simulink model "controllo_Completo_v14"  (R2025a)
settings: Solver=VariableStepAuto  StartTime=0.0  StopTime=Durata_Simulazione  MaxStep=Passo_integrazione_massimo  RelTol=1e-3
values from neighbouring files (symbols this model uses):
  C_bat_eq_rx = 1.0    (= 1)    [p_schema_completo_generale_v2.m]
  C_bat_eq_tx = 3.5    [p_schema_completo_generale_v2.m]
  C_bus_dc_dc = 1.5e-3    (= 0.0015)    [p_schema_completo_generale_v2.m]
  C_ris = 1/(w_dc_ac_nom^2*L_coil)    (= 6.49245057301e-08)    [p_schema_completo_generale_v2.m]
  dead_time_dc_dc = 0.3e-6    (= 3e-07)    [p_schema_completo_generale_v2.m]
  duty_A_0_tx = V_bat_0_tx/V_dc_0_tx    (= 0.472727272727)    [p_schema_completo_generale_v2.m]
  duty_B_0_tx = duty_A_0_tx    (= 0.472727272727)    [p_schema_completo_generale_v2.m]
  duty_leg_A_dc_dc_0_tx = V_bat_0_tx/V_dc_0_tx    (= 0.472727272727)    [p_schema_completo_generale_v2.m]
  duty_leg_B_dc_dc_0_tx = duty_leg_A_dc_dc_0_tx    (= 0.472727272727)    [p_schema_completo_generale_v2.m]
  Ibat_rif_max = 50    [p_schema_completo_generale_v2.m]
  Ibat_rif_min = -50    [p_schema_completo_generale_v2.m]
  Kp_P_tensione_batteria_rx = 1/modulo_catena_aperta_tensione_batteria_reg_P_rx    [p_schema_completo_generale_v2.m]
  Kp_P_tensione_batteria_tx = 1/modulo_catena_aperta_tensione_batteria_reg_P_tx    [p_schema_completo_generale_v2.m]
  L_coil = 54e-6    (= 5.4e-05)    [p_schema_completo_generale_v2.m]
  L_filtro_dc_dc = 65e-6    (= 6.5e-05)    [p_schema_completo_generale_v2.m]
  M_coil = k*sqrt(L_coil^2)    [p_schema_completo_generale_v2.m]
  Parametri_Controllori = [Parametri_Controllori     PI_corrente_trasm_tf_disc_den(2) PI_corrente_trasm_tf_disc_num(1) PI_corrente_trasm_tf_disc_num(2)]    [p_schema_completo_generale_v2.m]
  R_bat = 32e-3    (= 0.032)    [p_schema_completo_generale_v2.m]
  R_coil = w_dc_ac_nom*L_coil/Q_coil    (= 0.2883982056)    [p_schema_completo_generale_v2.m]
  R_coil_M = sqrt(w_dc_ac_nom^2)*M_coil/sqrt(Q_coil^2)    [p_schema_completo_generale_v2.m]
  R_Lfiltro_dc_dc = 6.5e-3    (= 0.0065)    [p_schema_completo_generale_v2.m]
  Req_Lfiltro_dc_dc = (R_Lfiltro_dc_dc+Rds_on_dc_dc)    (= 0.0075)    [p_schema_completo_generale_v2.m]
  Rshunt_coil = 1e5    (= 100000)    [p_schema_completo_generale_v2.m]
  Rshunt_Lfiltro = 1e6    (= 1000000)    [p_schema_completo_generale_v2.m]
  T_dc_ac = 1/freq_dc_ac    (= 1.17647058824e-05)    [p_schema_completo_generale_v2.m]
  T_dc_dc = 1/freq_dc_dc    (= 7.8431372549e-06)    [p_schema_completo_generale_v2.m]
  tau_filtro_anti_aliasing = R_filtro_anti_aliasing*C_filtro_anti_aliasing    (= 1.96e-06)    [p_schema_completo_generale_v2.m]
  tau_filtro_pb_coil = 1/(2*pi*f_filtro_pb_coil)    (= 3.18309886184e-05)    [p_schema_completo_generale_v2.m]
  tau_filtro_pb_corrente_bat = 1/(2*pi*f_filtro_pb_corrente_bat)    (= 2.49654812693e-05)    [p_schema_completo_generale_v2.m]
  Ts_BMS = 1e-3    (= 0.001)    [p_schema_completo_generale_v2.m]
  Ts_dc_ac = 4*T_dc_ac    (= 4.70588235294e-05)    [p_schema_completo_generale_v2.m]
  Ts_dc_dc = Ts_dc_ac    (= 4.70588235294e-05)    [p_schema_completo_generale_v2.m]
  Ts_trasmissione = 1e-3    (= 0.001)    [p_schema_completo_generale_v2.m]
  V_bat_0_rx = V_bat_nom    (= 96)    [p_schema_completo_generale_v2.m]
  V_bat_0_tx = V_bat_max-5    (= 104)    [p_schema_completo_generale_v2.m]
  V_bat_max = 109    [p_schema_completo_generale_v2.m]
  V_bat_max_alg = 218    [Controllo_tensione_bus_dc.m]    (also in Controllo_tensione_bus_dc_corrente_bobina.m; p_schema_completo_generale_v2.m)
  V_bat_min = 75    [p_schema_completo_generale_v2.m]
  V_bat_min_alg = 37.5    [Controllo_tensione_bus_dc.m]    (also in Controllo_tensione_bus_dc_corrente_bobina.m; p_schema_completo_generale_v2.m)
  V_dc_0_rx = 230    [p_schema_completo_generale_v2.m]
  V_dc_0_tx = 220    [p_schema_completo_generale_v2.m]
  Vbat_rif_max_tx = V_bat_max    (= 109)    [p_schema_completo_generale_v2.m]
  Vbat_rif_min_tx = V_bat_min    (= 75)    [p_schema_completo_generale_v2.m]
  Vdc_rif_max_tx = V_dc_nom+5    (= 255)    [p_schema_completo_generale_v2.m]
  Vdc_rif_min_tx = V_dc_nom-5    (= 245)    [p_schema_completo_generale_v2.m]
undefined symbols (not defined in the file or in its folder): Ceq_bat_tx, Cris_tx, Lfilt_dc_dc, Lfiltro_dc_dc_tx, R_bat_rx, R_bat_tx
libraries: simulink x44, spsSeriesRLCBranchLib x36, spsCurrentMeasurementLib x20, spsMosfetLib x16, spsVoltageMeasurementLib x12, simulink_extras x4, spsControlledCurrentSourceLib x4, spsControlledVoltageSourceLib x4, spsDCVoltageSourceLib x2, spsMutualInductanceLib x1, spsGroundLib x1, sps_lib x1
(part 1 of 7)
settings Model: Creator=bertman38930  LastModifiedBy=bertman38930
settings SolverCC: ZeroCrossAlgorithm=Adaptive
settings DebuggingCC: IgnoredZcDiagnostic=none

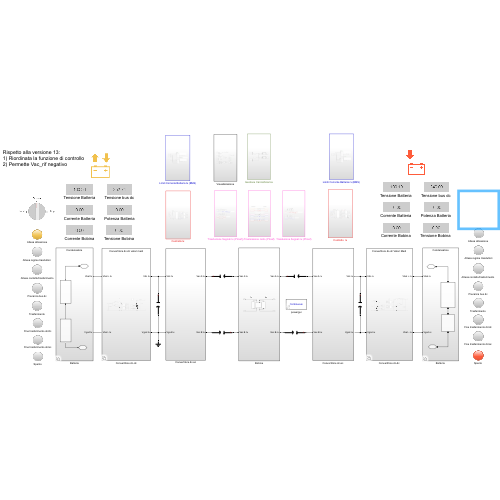
[thumbnail: Simulink's stored preview of the top-level diagram]
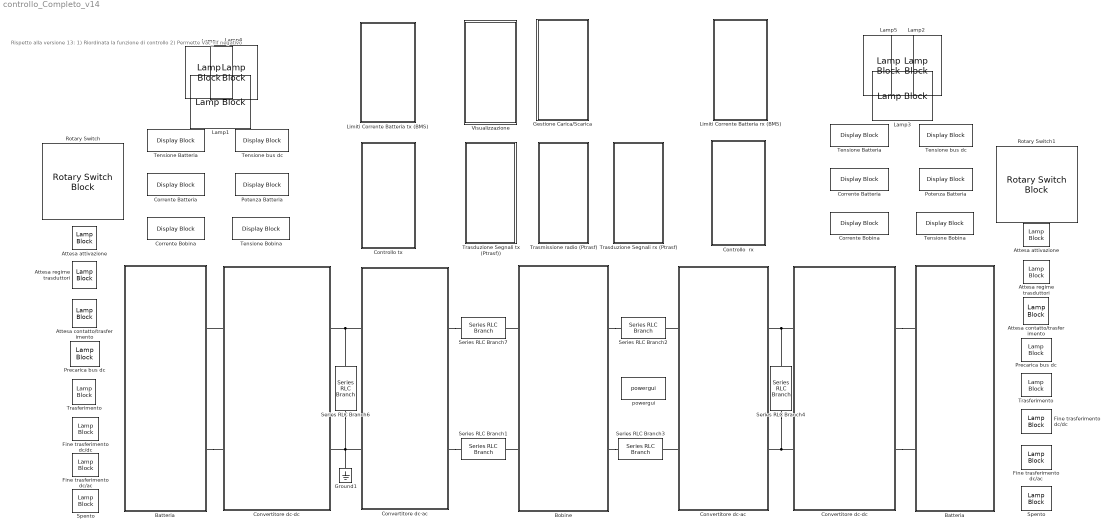
== system controllo_Completo_v14 ==
  note: Rispetto alla versione 13:
      | 1) Riordinata la funzione di controllo
      | 2) Permette Vac_rif negativo
  Attesa attivazione : LampBlock  LabelPosition=Hide  DefaultColor=[192.0, 192.0, 192.0]
  "Attesa attivazione " : LampBlock  LabelPosition=Hide  DefaultColor=[192.0, 192.0, 192.0]
  Attesa contatto/trasferimento : LampBlock  LabelPosition=Hide  DefaultColor=[192.0, 192.0, 192.0]
  "Attesa contatto/trasferimento " : LampBlock  LabelPosition=Hide  DefaultColor=[192.0, 192.0, 192.0]
  Attesa regime trasduttori : LampBlock  LabelPosition=Hide  DefaultColor=[192.0, 192.0, 192.0]
  "Attesa regime trasduttori " : LampBlock  LabelPosition=Hide  DefaultColor=[192.0, 192.0, 192.0]
  Batteria : Subsystem  Variant=on
  "Batteria " : Subsystem  Variant=on
  Bobine : Subsystem
  Controllo  rx : Subsystem
  Controllo tx : Subsystem
  Convertitore dc-ac : Subsystem  VariantControl=Selettore_Switching_0_Valori_Medi_1_dc_ac_tx==0
  "Convertitore dc-ac " : Subsystem  VariantControl=Selettore_Switching_0_Valori_Medi_1_dc_ac_rx==0
  Convertitore dc-dc : Subsystem  Variant=on
  "Convertitore dc-dc " : Subsystem  Variant=on
  Corrente Batteria : DisplayBlock  LabelPosition=Hide  Format=Custom  Transparency=1  FormatString=%.2f  GridColor=[0.502, 0.502, 0.502]
  "Corrente Batteria " : DisplayBlock  LabelPosition=Hide  Format=Custom  Transparency=1  FormatString=%.2f  GridColor=[0.502, 0.502, 0.502]
  Corrente Bobina : DisplayBlock  LabelPosition=Hide  Format=Custom  Transparency=1  FormatString=%.2f  GridColor=[0.502, 0.502, 0.502]
  "Corrente Bobina " : DisplayBlock  LabelPosition=Hide  Format=Custom  Transparency=1  FormatString=%.2f  GridColor=[0.502, 0.502, 0.502]
  Fine trasferimento dc/ac : LampBlock  LabelPosition=Hide  DefaultColor=[192.0, 192.0, 192.0]
  "Fine trasferimento dc/ac " : LampBlock  LabelPosition=Hide  DefaultColor=[192.0, 192.0, 192.0]
  Fine trasferimento dc/dc : LampBlock  LabelPosition=Hide  DefaultColor=[192.0, 192.0, 192.0]
  "Fine trasferimento dc/dc " : LampBlock  LabelPosition=Hide  DefaultColor=[192.0, 192.0, 192.0]
  Gestione Carica/Scarica : Subsystem
  Ground1 : spsGroundLib/Ground  LConnTagsString=a
  Lamp : LampBlock  LabelPosition=Hide  DefaultColor=[237.0, 177.0, 32.0]  Icon=TurnSignalLeft
  Lamp1 : LampBlock  LabelPosition=Hide  DefaultColor=[237.0, 177.0, 32.0]  Icon=Battery
  Lamp2 : LampBlock  LabelPosition=Hide  DefaultColor=[237.0, 177.0, 32.0]  Icon=TurnSignalRight
  Lamp3 : LampBlock  LabelPosition=Hide  DefaultColor=[237.0, 177.0, 32.0]  Icon=Battery
  Lamp4 : LampBlock  LabelPosition=Hide  DefaultColor=[237.0, 177.0, 32.0]  Icon=TurnSignalRight
  Lamp5 : LampBlock  LabelPosition=Hide  DefaultColor=[237.0, 177.0, 32.0]  Icon=TurnSignalRight
  Limiti Corrente Batteria rx (BMS) : Subsystem
  Limiti Corrente Batteria tx (BMS) : Subsystem
  Potenza Batteria : DisplayBlock  LabelPosition=Hide  Format=Custom  Transparency=1  FormatString=%.2f  GridColor=[0.502, 0.502, 0.502]
  "Potenza Batteria " : DisplayBlock  LabelPosition=Hide  Format=Custom  Transparency=1  FormatString=%.2f  GridColor=[0.502, 0.502, 0.502]
  Precarica bus dc : LampBlock  LabelPosition=Hide  DefaultColor=[192.0, 192.0, 192.0]
  "Precarica bus dc " : LampBlock  LabelPosition=Hide  DefaultColor=[192.0, 192.0, 192.0]
  Rotary Switch : RotarySwitchBlock  LabelPosition=Hide
  Rotary Switch1 : RotarySwitchBlock  LabelPosition=Hide
  Series RLC Branch1 : spsSeriesRLCBranchLib/Series RLC Branch  LConnTagsString=__new0  RConnTagsString=__new0  BranchType=C  Resistance=1  Inductance=Lfilt_dc_dc  SetiL0=off  InitialCurrent=0  Capacitance=C_ris*2  Setx0=off  InitialVoltage=V_Cfilter_tx_0  Measurements=None
  Series RLC Branch2 : spsSeriesRLCBranchLib/Series RLC Branch  LConnTagsString=__new0  RConnTagsString=__new0  BranchType=C  Resistance=1  Inductance=Lfilt_dc_dc  SetiL0=off  InitialCurrent=0  Capacitance=C_ris*2  Setx0=off  InitialVoltage=0  Measurements=None
  Series RLC Branch3 : spsSeriesRLCBranchLib/Series RLC Branch  LConnTagsString=__new0  RConnTagsString=__new0  BranchType=C  Resistance=1  Inductance=Lfilt_dc_dc  SetiL0=off  InitialCurrent=0  Capacitance=C_ris*2  Setx0=off  InitialVoltage=V_Cfilter_tx_0  Measurements=None
  Series RLC Branch4 : spsSeriesRLCBranchLib/Series RLC Branch  LConnTagsString=__new0  RConnTagsString=__new0  BranchType=C  Resistance=1  Inductance=Lfilt_dc_dc  SetiL0=off  InitialCurrent=0  Capacitance=C_bus_dc_dc  Setx0=on  InitialVoltage=V_dc_0_rx  Measurements=None
  Series RLC Branch6 : spsSeriesRLCBranchLib/Series RLC Branch  LConnTagsString=__new0  RConnTagsString=__new0  BranchType=C  Resistance=1  Inductance=Lfilt_dc_dc  SetiL0=off  InitialCurrent=0  Capacitance=C_bus_dc_dc  Setx0=on  InitialVoltage=V_dc_0_tx  Measurements=None
  Series RLC Branch7 : spsSeriesRLCBranchLib/Series RLC Branch  LConnTagsString=__new0  RConnTagsString=__new0  BranchType=C  Resistance=1  Inductance=Lfilt_dc_dc  SetiL0=off  InitialCurrent=0  Capacitance=C_ris*2  Setx0=off  InitialVoltage=V_Cfilter_tx_0  Measurements=None
  Spento : LampBlock  LabelPosition=Hide  DefaultColor=[192.0, 192.0, 192.0]
  "Spento " : LampBlock  LabelPosition=Hide  DefaultColor=[192.0, 192.0, 192.0]
  Tensione Batteria : DisplayBlock  LabelPosition=Hide  Format=Custom  Transparency=1  FormatString=%.2f  GridColor=[0.502, 0.502, 0.502]
  "Tensione Batteria " : DisplayBlock  LabelPosition=Hide  Format=Custom  Transparency=1  FormatString=%.2f  GridColor=[0.502, 0.502, 0.502]
  Tensione Bobina : DisplayBlock  LabelPosition=Hide  Format=Custom  Transparency=1  FormatString=%.2f  GridColor=[0.502, 0.502, 0.502]
  "Tensione Bobina " : DisplayBlock  LabelPosition=Hide  Format=Custom  Transparency=1  FormatString=%.2f  GridColor=[0.502, 0.502, 0.502]
  Tensione bus dc : DisplayBlock  LabelPosition=Hide  Format=Custom  Transparency=1  FormatString=%.2f  GridColor=[0.502, 0.502, 0.502]
  "Tensione bus dc " : DisplayBlock  LabelPosition=Hide  Format=Custom  Transparency=1  FormatString=%.2f  GridColor=[0.502, 0.502, 0.502]
  Trasduzione Segnali rx (Ptrasf) : Subsystem
  Trasduzione Segnali tx (Ptrasf)) : Subsystem
  Trasferimento : LampBlock  LabelPosition=Hide  DefaultColor=[192.0, 192.0, 192.0]
  "Trasferimento " : LampBlock  LabelPosition=Hide  DefaultColor=[192.0, 192.0, 192.0]
  Trasmissione radio (Ptrasf) : Subsystem
  Visualizzazione : Subsystem
  powergui : sps_lib/powergui  Priority=1  SimulationMode=Continuous  SampleTime=50e-6  frequency=60  Iterations=50  frequencyindice=0  Pbase=100e6  ErrMax=1e-4  UnitsV=kV  UnitsW=MW  buscounter=0  FunctionMessages=off  echomessages=off  EnableUseOfTLC=off  CurrentSourceSwitches=off  DisableSnubberDevices=off  DisableRonSwitches=off  DisableVfSwitches=off  DisplayEquations=off  AutomaticDiscreteSolvers=off  SolverType=Tustin/Backward Euler (TBE)  Interpol=off  ExternalGateDelay=off  methode=off  Ts=100  x0status=blocks  SPID=on  SwTol=0  HookPort=off  NonlinearTolerance=1e-4  nMaxIteration=100  ContinueOnMaxIteration=off  RestoreLinks=warning  ResistiveCurrentMeasurement=off  Frange=[0:2:500]  Ylog=off  Xlog=on  ShowGrid=off  save=off  variable=ZData  structure=0  ZoomFFT=off  StartTime=0.0  cycles=1  DisplayStyle=1  fundamental=60  FreqAxis=off  MaxFrequency=1000  frequencyindicesteady=1  RmsSteady=1  display=off
  connections:
  Series RLC Branch6/LConn1 -- Convertitore dc-ac/LConn1 -- Convertitore dc-dc/RConn1
  Series RLC Branch4/LConn1 -- "Convertitore dc-ac "/LConn1 -- "Convertitore dc-dc "/LConn1
  Series RLC Branch4/RConn1 -- "Convertitore dc-ac "/LConn2 -- "Convertitore dc-dc "/LConn2
  "Convertitore dc-ac "/RConn1 -- Series RLC Branch2/RConn1
  Bobine/RConn1 -- Series RLC Branch2/LConn1
  Bobine/LConn1 -- Series RLC Branch7/RConn1
  Bobine/LConn2 -- Series RLC Branch1/LConn1
  Convertitore dc-ac/RConn2 -- Series RLC Branch1/RConn1
  Convertitore dc-ac/RConn1 -- Series RLC Branch7/LConn1
  "Convertitore dc-ac "/RConn2 -- Series RLC Branch3/LConn1
  Bobine/RConn2 -- Series RLC Branch3/RConn1
  "Convertitore dc-dc "/RConn2 -- "Batteria "/RConn2
  "Convertitore dc-dc "/RConn1 -- "Batteria "/RConn1
  Convertitore dc-ac/LConn2 -- Ground1/LConn1 -- Series RLC Branch6/RConn1 -- Convertitore dc-dc/RConn2
  Batteria/RConn2 -- Convertitore dc-dc/LConn2
  Convertitore dc-dc/LConn1 -- Batteria/RConn1

== system controllo_Completo_v14/Batteria ==
  Batteria : Subsystem  VariantControl=Selettore_bat_Batteria_0_Condensatore_1_tx==0
  Condensatore : Subsystem  VariantControl=Selettore_bat_Batteria_0_Condensatore_1_tx==1
  Vbat tx : PMIOPort  Side=Right
  Vgnd tx : PMIOPort  Port=2  Side=Right

== system controllo_Completo_v14/Batteria  ==
  Batteria : Subsystem  VariantControl=Selettore_bat_Batteria_0_Condensatore_1_rx==0
  Condensatore : Subsystem  VariantControl=Selettore_bat_Batteria_0_Condensatore_1_rx==1
  Vbat rx : PMIOPort  Side=Right
  Vgnd rx : PMIOPort  Port=2  Side=Right

== system controllo_Completo_v14/Bobine ==
  note: Rx
  note: Tx
  Mutual Inductance : spsMutualInductanceLib/Mutual Inductance  LConnTagsString=a|b  RConnTagsString=A|B  TypeOfMutual=Two or three windings with equal mutual terms  NumberOfWindings=3  SelfImpedance1=[R_coil L_coil]  SelfImpedance2=[R_coil L_coil]  ThreeWindings=off  SelfImpedance3=[ 1.1 1.1e-03]  MutualImpedance=[R_coil_M M_coil]  InductanceMatrix="[1.0 0.9  0.9 ;  0.9 1.0  0.9;  0.9 0.9 1.0 ] * 1e-3"  ResistanceMatrix="[1.0 0.9  0.9 ;  0.9 1.0  0.9;  0.9 0.9 1.0 ]"  Measurements=None
      settings: LibrarySourceBlock=sps_lib/Passives/Mutual Inductance
  Series RLC Branch5 : spsSeriesRLCBranchLib/Series RLC Branch  LConnTagsString=__new0  RConnTagsString=__new0  BranchType=R  Resistance=Rshunt_coil  Inductance=Lfilt_dc_dc  SetiL0=off  InitialCurrent=0  Capacitance=Cris_tx*2  Setx0=off  InitialVoltage=V_Cfilter_tx_0  Measurements=None
  Series RLC Branch8 : spsSeriesRLCBranchLib/Series RLC Branch  LConnTagsString=__new0  RConnTagsString=__new0  BranchType=R  Resistance=Rshunt_coil  Inductance=Lfilt_dc_dc  SetiL0=off  InitialCurrent=0  Capacitance=Cris_tx*2  Setx0=off  InitialVoltage=V_Cfilter_tx_0  Measurements=None
  Vac A tx : PMIOPort  Side=Left
  Vac B tx : PMIOPort  Port=2  Side=Left
  Vac A rx : PMIOPort  Port=3  Side=Right
  Vac B rx : PMIOPort  Port=4  Side=Right
  connections:
  Series RLC Branch8/LConn1 -- Vac A rx/RConn1 -- Mutual Inductance/LConn2
  Series RLC Branch5/RConn1 -- Vac B tx/RConn1 -- Mutual Inductance/RConn1
  Series RLC Branch5/LConn1 -- Vac A tx/RConn1 -- Mutual Inductance/LConn1
  Mutual Inductance/RConn2 -- Vac B rx/RConn1 -- Series RLC Branch8/RConn1

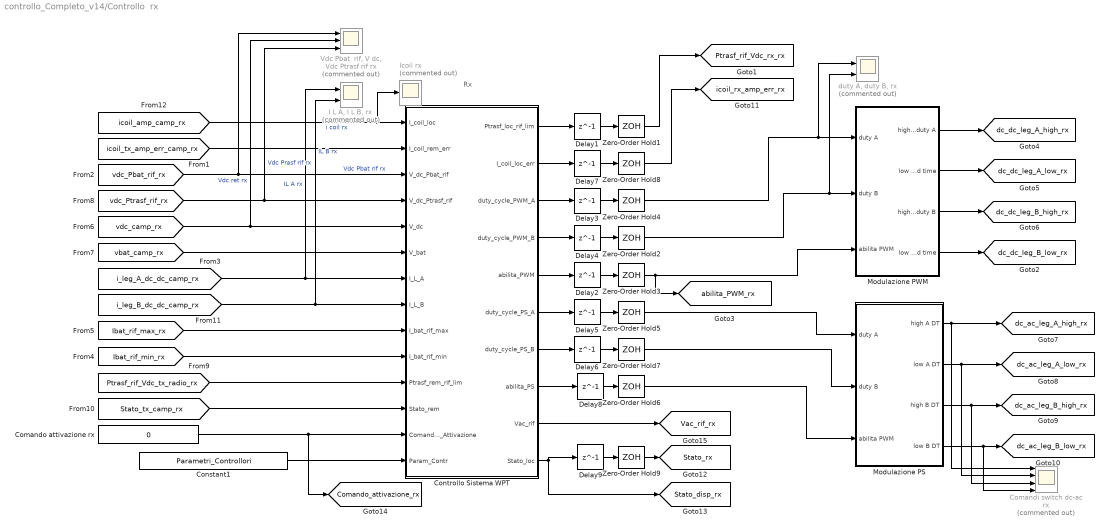
== system controllo_Completo_v14/Controllo  rx ==
  note: Rx
  Comandi switch dc-ac rx : Scope  Commented=on  NumInputPorts=4
      settings: ActiveDisplayYMinimum=-0.12499999999999997  ActiveDisplayYMaximum=1.125  DataLoggingDecimation=10  DataLoggingVariableName=ScopeData38
  Comando attivazione rx : Constant  Value=0
  Constant1 : Constant  Value=Parametri_Controllori
  Controllo Sistema WPT : MATLAB Function  TreatAsAtomicUnit=on  SystemSampleTime=Ts_dc_dc
  Delay1 : Delay  DelayLength=1  InitialCondition=0  SampleTime=Ts_dc_ac
  Delay2 : Delay  DelayLength=1  InitialCondition=0  SampleTime=Ts_dc_dc
  Delay3 : Delay  DelayLength=1  InitialCondition=duty_A_0_tx  SampleTime=Ts_dc_dc
  Delay4 : Delay  DelayLength=1  InitialCondition=duty_B_0_tx  SampleTime=Ts_dc_dc
  Delay5 : Delay  DelayLength=1  InitialCondition=0.5  SampleTime=Ts_dc_ac
  Delay6 : Delay  DelayLength=1  InitialCondition=0.5  SampleTime=Ts_dc_ac
  Delay7 : Delay  DelayLength=1  InitialCondition=0  SampleTime=Ts_dc_ac
  Delay8 : Delay  DelayLength=1  InitialCondition=0  SampleTime=Ts_dc_ac
  Delay9 : Delay  DelayLength=1  InitialCondition=0  SampleTime=Ts_dc_dc
  "I L A, I L B, rx" : Scope  Commented=on  NumInputPorts=2
      settings: ActiveDisplayYMinimum=-3.4060271798853266  ActiveDisplayYMaximum=0.37844746443173416  DataLoggingDecimation=10  DataLoggingVariableName=ScopeData21
  Icoil rx : Scope  Commented=on
      settings: ActiveDisplayYMinimum=-0.64051011286527737  ActiveDisplayYMaximum=5.7645910157874969  DataLoggingDecimation=10  DataLoggingVariableName=ScopeData9
  Modulazione PS : Subsystem
  Modulazione PWM : Subsystem
  "Vdc Pbat  rif, V dc, Vdc Ptrasf rif rx" : Scope  Commented=on  NumInputPorts=3
      settings: ActiveDisplayYMinimum=223.87602303237898  ActiveDisplayYMaximum=301.10375576550877  DataLoggingDecimation=10  DataLoggingVariableName=ScopeData4
  Zero-Order Hold{1,6..8} (4 alike) : ZeroOrderHold  SampleTime=Ts_dc_ac
  Zero-Order Hold{2..5,9} (5 alike) : ZeroOrderHold  SampleTime=Ts_dc_dc
  "duty A, duty B, rx" : Scope  Commented=on  NumInputPorts=2
      settings: ActiveDisplayYMinimum=-1.25  ActiveDisplayYMaximum=1.25  DataLoggingDecimation=10  DataLoggingVariableName=ScopeData40
  tag scope: Comando_attivazione_rx=global, Ptrasf_rif_Vdc_rx_rx=global, Stato_disp_rx=global, Stato_rx=global, Vac_rif_rx=global, abilita_PWM_rx=global, dc_ac_leg_A_high_rx=global, dc_ac_leg_A_low_rx=global, dc_ac_leg_B_high_rx=global, dc_ac_leg_B_low_rx=global, dc_dc_leg_A_high_rx=global, dc_dc_leg_A_low_rx=global, dc_dc_leg_B_high_rx=global, dc_dc_leg_B_low_rx=global, icoil_rx_amp_err_rx=global
  wires:
  Zero-Order Hold5/1 -> Modulazione PS/1(duty A)
  Zero-Order Hold7/1 -> Modulazione PS/2(duty B)
  Controllo Sistema WPT/8(abilita_PS) -> Delay8/1
  Zero-Order Hold8/1 -> [icoil_rx_amp_err_rx]
  Delay7/1 -> Zero-Order Hold8/1
  Delay6/1 -> Zero-Order Hold7/1
  Controllo Sistema WPT/7(duty_cycle_PS_B) -> Delay6/1
  Controllo Sistema WPT/6(duty_cycle_PS_A) -> Delay5/1
  Delay5/1 -> Zero-Order Hold5/1
  [Ibat_rif_max_rx] -> Controllo Sistema WPT/9(I_bat_rif_max)
  [vbat_camp_rx] -> Controllo Sistema WPT/6(V_bat)
  [i_leg_A_dc_dc_camp_rx] -> "I L A, I L B, rx"/1, Controllo Sistema WPT/7(I_L_A)  "IL A rx"
  Delay3/1 -> Zero-Order Hold4/1
  Delay4/1 -> Zero-Order Hold2/1
  Controllo Sistema WPT/3(duty_cycle_PWM_A) -> Delay3/1
  [Ibat_rif_min_rx] -> Controllo Sistema WPT/10(I_bat_rif_min)
  Controllo Sistema WPT/4(duty_cycle_PWM_B) -> Delay4/1
  [vdc_Pbat_rif_rx] -> "Vdc Pbat  rif, V dc, Vdc Ptrasf rif rx"/1, Controllo Sistema WPT/3(V_dc_Pbat_rif)  "Vdc Pbat rif rx"
  [i_leg_B_dc_dc_camp_rx] -> "I L A, I L B, rx"/2, Controllo Sistema WPT/8(I_L_B)  "IL B rx"
  Zero-Order Hold2/1 -> "duty A, duty B, rx"/2, Modulazione PWM/2(duty B)
  Modulazione PWM/1(high A dead time / duty A) -> [dc_dc_leg_A_high_rx]
  [vdc_camp_rx] -> Controllo Sistema WPT/5(V_dc), "Vdc Pbat  rif, V dc, Vdc Ptrasf rif rx"/2  "Vdc ret rx"
  Modulazione PWM/4(low B dead time) -> [dc_dc_leg_B_low_rx]
  Modulazione PWM/3(high B dead time / duty B) -> [dc_dc_leg_B_high_rx]
  Controllo Sistema WPT/5(abilita_PWM) -> Delay2/1
  Zero-Order Hold4/1 -> "duty A, duty B, rx"/1, Modulazione PWM/1(duty A)
  Modulazione PWM/2(low A dead time) -> [dc_dc_leg_A_low_rx]
  [icoil_tx_amp_err_camp_rx] -> Controllo Sistema WPT/2(I_coil_rem_err)
  Modulazione PS/1(high A DT) -> Comandi switch dc-ac rx/1, [dc_ac_leg_A_high_rx]
  Modulazione PS/4(low B DT) -> Comandi switch dc-ac rx/4, [dc_ac_leg_B_low_rx]
  Modulazione PS/3(high B DT) -> Comandi switch dc-ac rx/3, [dc_ac_leg_B_high_rx]
  Modulazione PS/2(low A DT) -> Comandi switch dc-ac rx/2, [dc_ac_leg_A_low_rx]
  [icoil_amp_camp_rx] -> Controllo Sistema WPT/1(I_coil_loc), Icoil rx/1  "i coil rx"
  Controllo Sistema WPT/2(I_coil_loc_err) -> Delay7/1
  [vdc_Ptrasf_rif_rx] -> "Vdc Pbat  rif, V dc, Vdc Ptrasf rif rx"/3, Controllo Sistema WPT/4(V_dc_Ptrasf_rif)  "Vdc Prasf rif rx"
  [Ptrasf_rif_Vdc_tx_radio_rx] -> Controllo Sistema WPT/11(Ptrasf_rem_rif_lim)
  Delay1/1 -> Zero-Order Hold1/1
  Zero-Order Hold1/1 -> [Ptrasf_rif_Vdc_rx_rx]
  Controllo Sistema WPT/1(Ptrasf_loc_rif_lim) -> Delay1/1
  Delay2/1 -> Zero-Order Hold3/1
  Zero-Order Hold3/1 -> Modulazione PWM/3(abilita PWM), [abilita_PWM_rx]
  Delay8/1 -> Zero-Order Hold6/1
  Zero-Order Hold6/1 -> Modulazione PS/3(abilita PWM)
  Constant1/1 -> Controllo Sistema WPT/14(Param_Contr)
  Controllo Sistema WPT/10(Stato_loc) -> Delay9/1, [Stato_disp_rx]
  Delay9/1 -> Zero-Order Hold9/1
  Zero-Order Hold9/1 -> [Stato_rx]
  [Stato_tx_camp_rx] -> Controllo Sistema WPT/12(Stato_rem)
  Comando attivazione rx/1 -> [Comando_attivazione_rx], Controllo Sistema WPT/13(Comando_Attivazione)
  Controllo Sistema WPT/9(Vac_rif) -> [Vac_rif_rx]

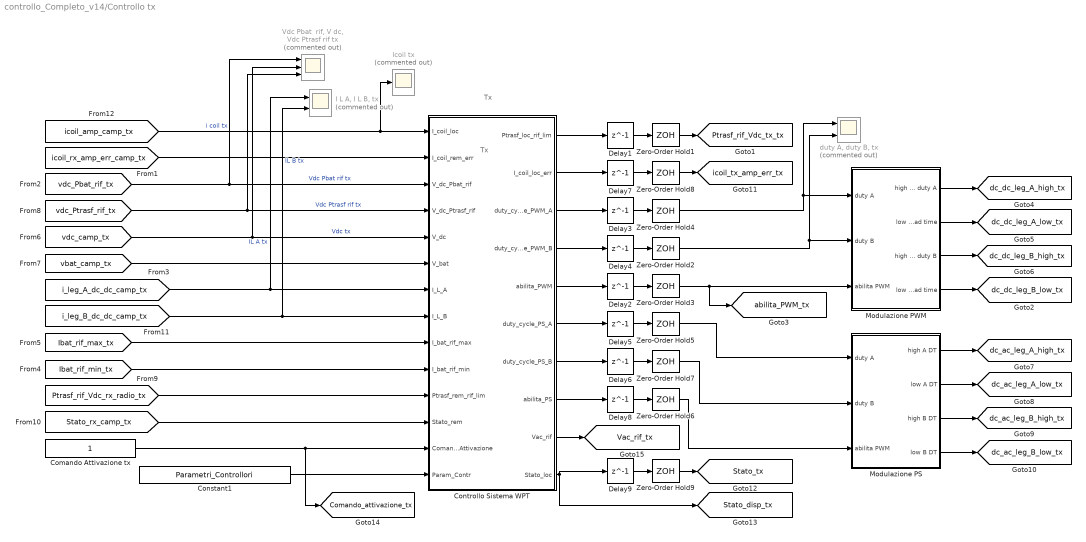
== system controllo_Completo_v14/Controllo tx ==
  note: Tx
  note: Tx
  Comando Attivazione tx : Constant
  Constant1 : Constant  Value=Parametri_Controllori
  Controllo Sistema WPT : MATLAB Function  TreatAsAtomicUnit=on  SystemSampleTime=Ts_dc_dc
  Delay1 : Delay  DelayLength=1  InitialCondition=0  SampleTime=Ts_dc_ac
  Delay2 : Delay  DelayLength=1  InitialCondition=0  SampleTime=Ts_dc_dc
  Delay3 : Delay  DelayLength=1  InitialCondition=duty_A_0_tx  SampleTime=Ts_dc_dc
  Delay4 : Delay  DelayLength=1  InitialCondition=duty_B_0_tx  SampleTime=Ts_dc_dc
  Delay5 : Delay  DelayLength=1  InitialCondition=0.5  SampleTime=Ts_dc_ac
  Delay6 : Delay  DelayLength=1  InitialCondition=0.5  SampleTime=Ts_dc_ac
  Delay7 : Delay  DelayLength=1  InitialCondition=0  SampleTime=Ts_dc_ac
  Delay8 : Delay  DelayLength=1  InitialCondition=0  SampleTime=Ts_dc_ac
  Delay9 : Delay  DelayLength=1  InitialCondition=0  SampleTime=Ts_dc_dc
  "I L A, I L B, tx" : Scope  Commented=on  NumInputPorts=2
      settings: ActiveDisplayYMinimum=-0.86085856605754507  ActiveDisplayYMaximum=7.7477263083146886  DataLoggingDecimation=10  DataLoggingVariableName=ScopeData21
  Icoil tx : Scope  Commented=on
      settings: ActiveDisplayYMinimum=-5.4935295857794459  ActiveDisplayYMaximum=49.441766272015023  DataLoggingDecimation=10  DataLoggingVariableName=ScopeData9
  Modulazione PS : Subsystem
  Modulazione PWM : Subsystem
  "Vdc Pbat  rif, V dc, Vdc Ptrasf rif tx" : Scope  Commented=on  NumInputPorts=3
      settings: ActiveDisplayYMinimum=-35.603873579228512  ActiveDisplayYMaximum=320.4348622130567  DataLoggingDecimation=10  DataLoggingVariableName=ScopeData7
  Zero-Order Hold{1,5..8} (5 alike) : ZeroOrderHold  SampleTime=Ts_dc_ac
  Zero-Order Hold{2..4,9} (4 alike) : ZeroOrderHold  SampleTime=Ts_dc_dc
  "duty A, duty B, tx" : Scope  Commented=on  NumInputPorts=2
      settings: ActiveDisplayYMinimum=-1.25  ActiveDisplayYMaximum=1.25  DataLoggingDecimation=10  DataLoggingVariableName=ScopeData40
  tag scope: Comando_attivazione_tx=global, Ptrasf_rif_Vdc_tx_tx=global, Stato_disp_tx=global, Stato_tx=global, Vac_rif_tx=global, abilita_PWM_tx=global, dc_ac_leg_A_high_tx=global, dc_ac_leg_A_low_tx=global, dc_ac_leg_B_high_tx=global, dc_ac_leg_B_low_tx=global, dc_dc_leg_A_high_tx=global, dc_dc_leg_A_low_tx=global, dc_dc_leg_B_high_tx=global, dc_dc_leg_B_low_tx=global, icoil_tx_amp_err_tx=global
  wires:
  [icoil_amp_camp_tx] -> Controllo Sistema WPT/1(I_coil_loc), Icoil tx/1  "i coil tx"
  Modulazione PS/2(low A DT) -> [dc_ac_leg_A_low_tx]
  Modulazione PS/3(high B DT) -> [dc_ac_leg_B_high_tx]
  Modulazione PS/4(low B DT) -> [dc_ac_leg_B_low_tx]
  Modulazione PS/1(high A DT) -> [dc_ac_leg_A_high_tx]
  [icoil_rx_amp_err_camp_tx] -> Controllo Sistema WPT/2(I_coil_rem_err)
  Modulazione PWM/2(low A dead time) -> [dc_dc_leg_A_low_tx]
  Zero-Order Hold4/1 -> "duty A, duty B, tx"/1, Modulazione PWM/1(duty A)
  Controllo Sistema WPT/5(abilita_PWM) -> Delay2/1
  Modulazione PWM/3(high B dead time / duty B) -> [dc_dc_leg_B_high_tx]
  Modulazione PWM/4(low B dead time) -> [dc_dc_leg_B_low_tx]
  [vdc_camp_tx] -> "Vdc Pbat  rif, V dc, Vdc Ptrasf rif tx"/2, Controllo Sistema WPT/5(V_dc)  "Vdc tx"
  Modulazione PWM/1(high A dead time / duty A) -> [dc_dc_leg_A_high_tx]
  Zero-Order Hold2/1 -> "duty A, duty B, tx"/2, Modulazione PWM/2(duty B)
  [i_leg_B_dc_dc_camp_tx] -> Controllo Sistema WPT/8(I_L_B), "I L A, I L B, tx"/2  "IL B tx"
  [vdc_Pbat_rif_tx] -> "Vdc Pbat  rif, V dc, Vdc Ptrasf rif tx"/1, Controllo Sistema WPT/3(V_dc_Pbat_rif)  "Vdc Pbat rif tx"
  Controllo Sistema WPT/4(duty_cycle_PWM_B) -> Delay4/1
  [Ibat_rif_min_tx] -> Controllo Sistema WPT/10(I_bat_rif_min)
  Controllo Sistema WPT/3(duty_cycle_PWM_A) -> Delay3/1
  Delay4/1 -> Zero-Order Hold2/1
  Delay3/1 -> Zero-Order Hold4/1
  [i_leg_A_dc_dc_camp_tx] -> Controllo Sistema WPT/7(I_L_A), "I L A, I L B, tx"/1  "IL A tx"
  [vbat_camp_tx] -> Controllo Sistema WPT/6(V_bat)
  [Ibat_rif_max_tx] -> Controllo Sistema WPT/9(I_bat_rif_max)
  Delay5/1 -> Zero-Order Hold5/1
  Controllo Sistema WPT/6(duty_cycle_PS_A) -> Delay5/1
  Controllo Sistema WPT/7(duty_cycle_PS_B) -> Delay6/1
  Delay6/1 -> Zero-Order Hold7/1
  Controllo Sistema WPT/2(I_coil_loc_err) -> Delay7/1
  Delay7/1 -> Zero-Order Hold8/1
  Zero-Order Hold8/1 -> [icoil_tx_amp_err_tx]
  Controllo Sistema WPT/8(abilita_PS) -> Delay8/1
  Zero-Order Hold7/1 -> Modulazione PS/2(duty B)
  Zero-Order Hold5/1 -> Modulazione PS/1(duty A)
  [vdc_Ptrasf_rif_tx] -> "Vdc Pbat  rif, V dc, Vdc Ptrasf rif tx"/3, Controllo Sistema WPT/4(V_dc_Ptrasf_rif)  "Vdc Ptrasf rif tx"
  [Ptrasf_rif_Vdc_rx_radio_tx] -> Controllo Sistema WPT/11(Ptrasf_rem_rif_lim)
  Controllo Sistema WPT/1(Ptrasf_loc_rif_lim) -> Delay1/1
  Delay1/1 -> Zero-Order Hold1/1
  Zero-Order Hold1/1 -> [Ptrasf_rif_Vdc_tx_tx]
  Delay2/1 -> Zero-Order Hold3/1
  Zero-Order Hold3/1 -> [abilita_PWM_tx], Modulazione PWM/3(abilita PWM)
  Delay8/1 -> Zero-Order Hold6/1
  Zero-Order Hold6/1 -> Modulazione PS/3(abilita PWM)
  Constant1/1 -> Controllo Sistema WPT/14(Param_Contr)
  Controllo Sistema WPT/10(Stato_loc) -> Delay9/1, [Stato_disp_tx]
  Delay9/1 -> Zero-Order Hold9/1
  Zero-Order Hold9/1 -> [Stato_tx]
  [Stato_rx_camp_tx] -> Controllo Sistema WPT/12(Stato_rem)
  Comando Attivazione tx/1 -> [Comando_attivazione_tx], Controllo Sistema WPT/13(Comando_Attivazione)
  Controllo Sistema WPT/9(Vac_rif) -> [Vac_rif_tx]

== system controllo_Completo_v14/Convertitore dc-ac ==
  note: Tx
  Current Measurement1 : spsCurrentMeasurementLib/Current Measurement  PhasorSimulation=off  OutputType=Complex  PSBequivalent=0
  Current Measurement3 : spsCurrentMeasurementLib/Current Measurement  PhasorSimulation=off  OutputType=Complex  PSBequivalent=0
  I coil tx : Scope  Commented=on
      settings: ActiveDisplayYMinimum=-77.357202499076465  ActiveDisplayYMaximum=77.357345547091711  DataLoggingVariableName=ScopeData35
  Mosfet{1..4} (4 alike) : spsMosfetLib/Mosfet  Ron=Rds_on_dc_ac  Lon=0  Rd=Ron_diodo_dc_ac  Vfd=Vf_diodo_dc_ac  IC=0  Rs=Rsnubber_dc_ac  Cs=Csnubber_dc_ac  Measurements=off
  Voltage Measurement : spsVoltageMeasurementLib/Voltage Measurement  PhasorSimulation=off  OutputType=Complex  PSBequivalent=0
  Voltage Measurement1 : spsVoltageMeasurementLib/Voltage Measurement  PhasorSimulation=off  OutputType=Complex  PSBequivalent=0
  v coil tx : Scope  Commented=on
      settings: ActiveDisplayYMinimum=-312.49999999999403  ActiveDisplayYMaximum=312.49999999999437  DataLoggingVariableName=ScopeData8
  Vdc tx : PMIOPort  Side=Left
  Vac A tx : PMIOPort  Port=2  Side=Right
  Vac B tx : PMIOPort  Port=3  Side=Right
  Vgnd tx : PMIOPort  Port=4  Side=Left
  tag scope: i_coil_tx=global, i_dc_ac_tx=global, v_coil_tx=global, v_dc_tx=global
  wires:
  [dc_ac_leg_B_high_tx] -> Mosfet1/1
  [dc_ac_leg_B_low_tx] -> Mosfet2/1
  [dc_ac_leg_A_low_tx] -> Mosfet3/1
  [dc_ac_leg_A_high_tx] -> Mosfet4/1
  Current Measurement3/1 -> [i_coil_tx], I coil tx/1
  Voltage Measurement/1 -> v coil tx/1, [v_coil_tx]  "v coil tx"
  Current Measurement1/1 -> [i_dc_ac_tx]
  Voltage Measurement1/1 -> [v_dc_tx]
  connections:
  Vac B tx/RConn1 -- Mosfet2/LConn1 -- Mosfet1/RConn1 -- Voltage Measurement/LConn2
  Voltage Measurement/LConn1 -- Mosfet3/LConn1 -- Mosfet4/RConn1 -- Current Measurement3/LConn1
  Current Measurement1/RConn1 -- Mosfet1/LConn1 -- Mosfet4/LConn1
  Mosfet3/RConn1 -- Mosfet2/RConn1 -- Voltage Measurement1/LConn2 -- Vgnd tx/RConn1
  Current Measurement3/RConn1 -- Vac A tx/RConn1
  Current Measurement1/LConn1 -- Voltage Measurement1/LConn1 -- Vdc tx/RConn1

== system controllo_Completo_v14/Convertitore dc-ac  ==
  note: Rx
  Current Measurement1 : spsCurrentMeasurementLib/Current Measurement  PhasorSimulation=off  OutputType=Complex  PSBequivalent=0
  Current Measurement3 : spsCurrentMeasurementLib/Current Measurement  PhasorSimulation=off  OutputType=Complex  PSBequivalent=0
  Mosfet{1..3,6} (4 alike) : spsMosfetLib/Mosfet  Ron=Rds_on_dc_ac  Lon=0  Rd=Ron_diodo_dc_ac  Vfd=Vf_diodo_dc_ac  IC=0  Rs=Rsnubber_dc_ac  Cs=Csnubber_dc_ac  Measurements=off
  Voltage Measurement : spsVoltageMeasurementLib/Voltage Measurement  PhasorSimulation=off  OutputType=Complex  PSBequivalent=0
  Voltage Measurement1 : spsVoltageMeasurementLib/Voltage Measurement  PhasorSimulation=off  OutputType=Complex  PSBequivalent=0
  i coil rx : Scope  Commented=on
      settings: ActiveDisplayYMinimum=-51.316027307256377  ActiveDisplayYMaximum=51.312748018112082  DataLoggingVariableName=ScopeData25
  v coil rx : Scope  Commented=on
      settings: ActiveDisplayYMinimum=-2.3978455036975813E+298  ActiveDisplayYMaximum=2.4051957397188807E+298  DataLoggingVariableName=ScopeData26
  Vdc rx : PMIOPort  Side=Left
  Vac A rx : PMIOPort  Port=2  Side=Right
  Vac B rx : PMIOPort  Port=3  Side=Right
  Vgnd rx : PMIOPort  Port=4  Side=Left
  tag scope: i_coil_rx=global, i_dc_ac_rx=global, v_coil_rx=global, v_dc_rx=global
  wires:
  Current Measurement1/1 -> [i_dc_ac_rx]
  Voltage Measurement1/1 -> [v_dc_rx]
  Voltage Measurement/1 -> [v_coil_rx], v coil rx/1
  [dc_ac_leg_B_high_rx] -> Mosfet6/1
  [dc_ac_leg_B_low_rx] -> Mosfet3/1
  [dc_ac_leg_A_low_rx] -> Mosfet2/1
  [dc_ac_leg_A_high_rx] -> Mosfet1/1
  Current Measurement3/1 -> [i_coil_rx], i coil rx/1
  connections:
  Current Measurement1/LConn1 -- Vdc rx/RConn1
  Voltage Measurement/LConn2 -- Mosfet3/LConn1 -- Vac B rx/RConn1 -- Mosfet6/RConn1
  Current Measurement3/LConn1 -- Mosfet1/RConn1 -- Mosfet2/LConn1 -- Voltage Measurement/LConn1
  Voltage Measurement1/LConn1 -- Current Measurement1/RConn1 -- Mosfet1/LConn1 -- Mosfet6/LConn1
  Vgnd rx/RConn1 -- Voltage Measurement1/LConn2 -- Mosfet3/RConn1 -- Mosfet2/RConn1
  Current Measurement3/RConn1 -- Vac A rx/RConn1

== system controllo_Completo_v14/Convertitore dc-dc ==
  note: Tx
  Convertitore dc-dc switching : Subsystem  VariantControl=Selettore_Switching_0_Valori_Medi_1_dc_dc_tx==0
  Convertitore dc-dc valori medi : Subsystem  VariantControl=Selettore_Switching_0_Valori_Medi_1_dc_dc_tx==1
  Vdc tx : PMIOPort  Side=Right
  Vbat + tx : PMIOPort  Port=2  Side=Left
  Vgnd tx : PMIOPort  Port=3  Side=Right
  Vbat - tx : PMIOPort  Port=4  Side=Left

== system controllo_Completo_v14/Convertitore dc-dc  ==
  note: Rx
  "Convertitore dc-dc Switching " : Subsystem  VariantControl=Selettore_Switching_0_Valori_Medi_1_dc_dc_rx==0
  "Convertitore dc-dc Valori Medi " : Subsystem  VariantControl=Selettore_Switching_0_Valori_Medi_1_dc_dc_rx==1
  Vdc rx : PMIOPort  Side=Left
  "Vgnd rx " : PMIOPort  Port=2  Side=Left
  Vbat + rx : PMIOPort  Port=3  Side=Right
  Vbat - rx : PMIOPort  Port=4  Side=Right

== system controllo_Completo_v14/Gestione Carica//Scarica ==
  Constant11 : Constant  Value=Vdc_rif_min_tx
  Constant12 : Constant  Value=Vbat_rif_max_tx
  Constant13 : Constant  Value=Vdc_rif_max_tx
  Constant3 : Constant  Value=Vdc_rif_max_tx
  Constant5 : Constant  Value=Vbat_rif_min_tx
  Constant8 : Constant  Value=Vdc_rif_min_tx
  Demux : Demux  Outputs=3
  Demux1 : Demux  Outputs=3
  Display{,1..5} (6 alike) : Display
  Mux : Mux  Inputs=3
  Mux1 : Mux  Inputs=3
  Switch : Switch  Criteria=u2 > Threshold  Threshold=0.5  SaturateOnIntegerOverflow=off  InputSameDT=off
  Switch1 : Switch  Criteria=u2 > Threshold  Threshold=0.5  SaturateOnIntegerOverflow=off  InputSameDT=off
  tag scope: Vbat_rif_rx=global, Vbat_rif_tx=global, vdc_Pbat_rif_rx=global, vdc_Pbat_rif_tx=global, vdc_Ptrasf_rif_rx=global, vdc_Ptrasf_rif_tx=global
  wires:
  Mux/1 -> Switch/1, Switch1/1
  Constant5/1 -> Mux/1
  Constant3/1 -> Mux/2
  Constant8/1 -> Mux/3
  Constant11/1 -> Mux1/2
  Constant13/1 -> Mux1/3
  Constant12/1 -> Mux1/1
  Mux1/1 -> Switch1/3, Switch/3
  Switch/1 -> Demux/1
  [Comando_attivazione_tx] -> Switch/2
  Demux/1 -> Display/1, [Vbat_rif_tx]
  Demux/2 -> Display1/1, [vdc_Pbat_rif_tx]
  Demux/3 -> [vdc_Ptrasf_rif_tx], Display2/1
  Demux1/3 -> [vdc_Ptrasf_rif_rx], Display5/1
  Demux1/2 -> Display4/1, [vdc_Pbat_rif_rx]
  Switch1/1 -> Demux1/1
  Demux1/1 -> Display3/1, [Vbat_rif_rx]
  [Comando_attivazione_rx] -> Switch1/2

== system controllo_Completo_v14/Limiti Corrente Batteria rx (BMS) ==
  note: Questo regolatore controlla la carica della batteria.
      | Tenta di portare la tensione al valore massimo e genera un riferimento per la corrente da scambiare con la batteria.
      | Secondo le convenzioni la corrente di carica della batteria è negativa per cui il riferimento di corrente generato sarà negativo.
      | La corrente scambiata con la batteria non può essere minore di questo riferimento altrimenti la batteria sarebbe sovraccaricata.
      | Dato che il riferimento di corrente è usato come limite per gli altri anelli di controllo ma non viene effettivamente applicato, è conveniente che il regolatore che lo genera sia di tipo P altrimenti si avrebbe il windup.
  note: Questo regolatore controlla la scarica della batteria.
      | Tenta di portare la tensione al valore minimo e genera un riferimento per la corrente da scambiare con la batteria.
      | Secondo le convenzioni la corrente di scarica della batteria è positiva per cui il riferimento di corrente generato sarà positivo.
      | La corrente scambiata con la batteria non può essere maggiore di questo riferimento altrimenti la batteria sarebbe scaricata troppo.
      | Dato che il riferimento di corrente è usato come limite per gli altri anelli di controllo ma non viene effettivamente applicato, è conveniente che il regolatore che lo genera sia di tipo P altrimenti si avrebbe il windup.
  Constant : Constant  Value=Ibat_rif_max
  Constant1 : Constant  Value=Ibat_rif_min
  Constant2 : Constant  Value=V_bat_max
  Constant3 : Constant  Value=V_bat_min
  Controllo carica bat tx : Subsystem
  Controllo scarica bat tx : Subsystem
  "Ibat rif min rx, Ibat rif max rx" : Scope  NumInputPorts=2
      settings: ActiveDisplayYMinimum=-62.500000000000007  ActiveDisplayYMaximum=62.500000000000007  DataLoggingDecimation=10  DataLoggingVariableName=ScopeData37
  Saturation1 : Saturate  UpperLimit=V_bat_max_alg  LowerLimit=V_bat_min_alg
  "Vbat max rx, Vbat ret rx, V bat min rx" : Scope  Commented=on  NumInputPorts=3
      settings: ActiveDisplayYMinimum=93.4132552385858  ActiveDisplayYMaximum=110.73186052904603  DataLoggingDecimation=10  DataLoggingVariableName=ScopeData18
  Zero-Order Hold{1..4} (4 alike) : ZeroOrderHold  SampleTime=Ts_BMS
  tag scope: Ibat_rif_max_rx=global, Ibat_rif_min_rx=global
  wires:
  Constant/1 -> Zero-Order Hold3/1
  Constant1/1 -> Zero-Order Hold4/1
  Zero-Order Hold3/1 -> Controllo scarica bat tx/3(Ibat rif max), Controllo carica bat tx/3(Ibat rif max)
  Zero-Order Hold4/1 -> Controllo scarica bat tx/4(I bat rif min), Controllo carica bat tx/4(I bat rif min)
  Controllo carica bat tx/1(Ibat rif rx) -> "Ibat rif min rx, Ibat rif max rx"/1, [Ibat_rif_min_rx]  "Ibat rif min rx"
  Zero-Order Hold2/1 -> "Vbat max rx, Vbat ret rx, V bat min rx"/1, Controllo carica bat tx/1(Vbat  rif)  "Vbat max rx"
  [vbat_camp_rx] -> Saturation1/1  "Vbat ret rx"
  Constant2/1 -> Zero-Order Hold2/1
  Constant3/1 -> Zero-Order Hold1/1
  Zero-Order Hold1/1 -> "Vbat max rx, Vbat ret rx, V bat min rx"/3, Controllo scarica bat tx/1(Vbat  rif)  "Vbat min rx"
  Controllo scarica bat tx/1(Ibat rif rx) -> "Ibat rif min rx, Ibat rif max rx"/2, [Ibat_rif_max_rx]  "Ibat rif max rx"
  Saturation1/1 -> Controllo scarica bat tx/2(Vbat), Controllo carica bat tx/2(Vbat), "Vbat max rx, Vbat ret rx, V bat min rx"/2

== system controllo_Completo_v14/Limiti Corrente Batteria tx (BMS) ==
  note: Questo regolatore controlla la carica della batteria.
      | Tenta di portare la tensione al valore massimo e genera un riferimento per la corrente da scambiare con la batteria.
      | Secondo le convenzioni la corrente di carica della batteria è negativa per cui il riferimento di corrente generato sarà negativo.
      | La corrente scambiata con la batteria non può essere minore di questo riferimento altrimenti la batteria sarebbe sovraccaricata.
      | Dato che il riferimento di corrente è usato come limite per gli altri anelli di controllo ma non viene effettivamente applicato, è conveniente che il regolatore che lo genera sia di tipo P altrimenti si avrebbe il windup.
  note: Questo regolatore controlla la scarica della batteria.
      | Tenta di portare la tensione al valore minimo e genera un riferimento per la corrente da scambiare con la batteria.
      | Secondo le convenzioni la corrente di scarica della batteria è positiva per cui il riferimento di corrente generato sarà positivo.
      | La corrente scambiata con la batteria non può essere maggiore di questo riferimento altrimenti la batteria sarebbe scaricata troppo.
      | Dato che il riferimento di corrente è usato come limite per gli altri anelli di controllo ma non viene effettivamente applicato, è conveniente che il regolatore che lo genera sia di tipo P altrimenti si avrebbe il windup.
  note: Gli anelli di controllo sono basati sulla manipolazione
      | dell potenza scambiata e quindi sarebbe stato più
      | logico generare dei limiti di potenza. Tuttavia spesso il
      | BMS fornisce dei limiti di carrente e quindi si è operato
      | in accordo a questo approccio in modo da rendere più
      | semplice l'implementazione del controll nel sistema reale
  Constant : Constant  Value=Ibat_rif_max
  Constant1 : Constant  Value=Ibat_rif_min
  Constant2 : Constant  Value=V_bat_max
  Constant3 : Constant  Value=V_bat_min
  Controllo carica bat tx : Subsystem
  Controllo scarica bat tx : Subsystem
  "Ibat rif min tx, Ibat rif max tc" : Scope  NumInputPorts=2
      settings: ActiveDisplayYMinimum=-62.500000000000007  ActiveDisplayYMaximum=62.500000000000007  DataLoggingDecimation=10  DataLoggingVariableName=ScopeData37
  Saturation1 : Saturate  UpperLimit=V_bat_max_alg  LowerLimit=V_bat_min_alg
  "Vbat max, ret, min tx" : Scope  Commented=on  NumInputPorts=3
      settings: ActiveDisplayYMinimum=31.150866018328603  ActiveDisplayYMaximum=120.5258660183286  DataLoggingDecimation=10  DataLoggingVariableName=ScopeData18
  Zero-Order Hold{1..4} (4 alike) : ZeroOrderHold  SampleTime=Ts_BMS
  tag scope: Ibat_rif_max_tx=global, Ibat_rif_min_tx=global
  wires:
  Constant/1 -> Zero-Order Hold3/1
  Constant1/1 -> Zero-Order Hold4/1
  Zero-Order Hold3/1 -> Controllo carica bat tx/3(Ibat rif max), Controllo scarica bat tx/3(Ibat rif max)
  Zero-Order Hold4/1 -> Controllo carica bat tx/4(I bat rif min), Controllo scarica bat tx/4(I bat rif min)
  Controllo carica bat tx/1(Ibat rif tx) -> "Ibat rif min tx, Ibat rif max tc"/1, [Ibat_rif_min_tx]  "Ibat rif min tx"
  Zero-Order Hold2/1 -> "Vbat max, ret, min tx"/1, Controllo carica bat tx/1(Vbat  rif)  "Vbat max tx"
  [vbat_camp_tx] -> Saturation1/1
  Constant2/1 -> Zero-Order Hold2/1
  Constant3/1 -> Zero-Order Hold1/1
  Zero-Order Hold1/1 -> "Vbat max, ret, min tx"/3, Controllo scarica bat tx/1(Vbat  rif)  "Vbat min tx"
  Controllo scarica bat tx/1(Ibat rif tx) -> "Ibat rif min tx, Ibat rif max tc"/2, [Ibat_rif_max_tx]  "Ibat rif max tx"
  Saturation1/1 -> Controllo carica bat tx/2(Vbat), "Vbat max, ret, min tx"/2, Controllo scarica bat tx/2(Vbat)  "Vbat ret tx"

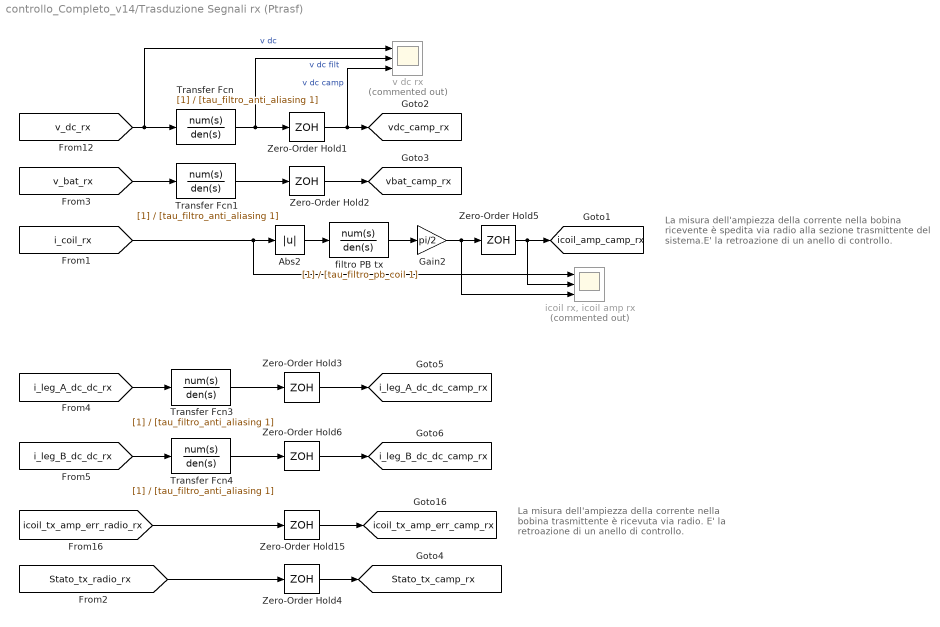
== system controllo_Completo_v14/Trasduzione Segnali rx (Ptrasf) ==
  note: La misura dell'ampiezza della corrente
      | nella bobina ricevente è spedita via radio
      | alla sezione trasmittente del sistema.E' la retroazione di
      | un anello di controllo.
  note: La misura dell'ampiezza della corrente
      | nella bobina trasmittente è ricevuta via radio.
      | E' la retroazione di un anello di controllo.
  Abs2 : Abs  SaturateOnIntegerOverflow=off
  Gain2 : Gain  Gain=pi/2
  Transfer Fcn{,1,3..4} (4 alike) : TransferFcn  Denominator=[tau_filtro_anti_aliasing 1]
  Zero-Order Hold{1..3,6} (4 alike) : ZeroOrderHold  SampleTime=Ts_dc_dc
  Zero-Order Hold15 : ZeroOrderHold  SampleTime=Ts_dc_ac
  Zero-Order Hold4 : ZeroOrderHold  SampleTime=Ts_dc_ac
  Zero-Order Hold5 : ZeroOrderHold  SampleTime=Ts_dc_ac
  filtro PB tx : TransferFcn  Denominator=[tau_filtro_pb_coil 1]
  "icoil rx, icoil amp rx" : Scope  Commented=on  NumInputPorts=3
      settings: ActiveDisplayYMinimum=-59.379349724833858  ActiveDisplayYMaximum=60.463969998037072  DataLoggingDecimation=10  DataLoggingVariableName=ScopeData27
  v dc rx : Scope  Commented=on  NumInputPorts=3
      settings: ActiveDisplayYMinimum=110.47319204966614  ActiveDisplayYMaximum=125.3410479176644  DataLoggingDecimation=10  DataLoggingVariableName=ScopeData19
  tag scope: Stato_tx_camp_rx=global, i_leg_A_dc_dc_camp_rx=global, i_leg_B_dc_dc_camp_rx=global, icoil_amp_camp_rx=global, icoil_tx_amp_err_camp_rx=global, vbat_camp_rx=global, vdc_camp_rx=global
  wires:
  Transfer Fcn4/1 -> Zero-Order Hold6/1
  Transfer Fcn3/1 -> Zero-Order Hold3/1
  Transfer Fcn1/1 -> Zero-Order Hold2/1
  Transfer Fcn/1 -> v dc rx/2, Zero-Order Hold1/1  "v dc filt"
  Zero-Order Hold15/1 -> [icoil_tx_amp_err_camp_rx]
  [icoil_tx_amp_err_radio_rx] -> Zero-Order Hold15/1
  [i_leg_B_dc_dc_rx] -> Transfer Fcn4/1
  Zero-Order Hold6/1 -> [i_leg_B_dc_dc_camp_rx]
  [i_leg_A_dc_dc_rx] -> Transfer Fcn3/1
  Zero-Order Hold3/1 -> [i_leg_A_dc_dc_camp_rx]
  filtro PB tx/1 -> Gain2/1
  Zero-Order Hold5/1 -> [icoil_amp_camp_rx], "icoil rx, icoil amp rx"/2
  Abs2/1 -> filtro PB tx/1
  [v_dc_rx] -> v dc rx/1, Transfer Fcn/1  "v dc"
  Zero-Order Hold1/1 -> v dc rx/3, [vdc_camp_rx]  "v dc camp"
  [v_bat_rx] -> Transfer Fcn1/1
  Zero-Order Hold2/1 -> [vbat_camp_rx]
  [i_coil_rx] -> Abs2/1, "icoil rx, icoil amp rx"/1
  [Stato_tx_radio_rx] -> Zero-Order Hold4/1
  Zero-Order Hold4/1 -> [Stato_tx_camp_rx]
  Gain2/1 -> "icoil rx, icoil amp rx"/3, Zero-Order Hold5/1

== system controllo_Completo_v14/Trasduzione Segnali tx (Ptrasf)) ==
  note: La misura dell'ampiezza della corrente
      | nella bobina ricevente è ricevuta via radio.
      | E' la retroazione di un anello di controllo.
  note: La misura dell'ampiezza della corrente
      | nella bobina trasmittente è spedita via radio
      | alla sezione ricevente del sistema.
      | E' la retroazione di un anello di controllo.
  Abs2 : Abs  SaturateOnIntegerOverflow=off
  Gain2 : Gain  Gain=pi/2
  Transfer Fcn{,1,3..4} (4 alike) : TransferFcn  Denominator=[tau_filtro_anti_aliasing 1]
  Zero-Order Hold{1..3,6} (4 alike) : ZeroOrderHold  SampleTime=Ts_dc_dc
  Zero-Order Hold4 : ZeroOrderHold  SampleTime=Ts_dc_ac
  Zero-Order Hold5 : ZeroOrderHold  SampleTime=Ts_dc_ac
  Zero-Order Hold8 : ZeroOrderHold  SampleTime=Ts_dc_ac
  filtro PB : TransferFcn  Denominator=[tau_filtro_pb_coil 1]
  "icoil tx, icoil amp tx" : Scope  Commented=on  NumInputPorts=3
      settings: ActiveDisplayYMinimum=-3.1442033838195016  ActiveDisplayYMaximum=3.1451564599272936  DataLoggingDecimation=10  DataLoggingVariableName=ScopeData28
  tag scope: Stato_rx_camp_tx=global, i_leg_A_dc_dc_camp_tx=global, i_leg_B_dc_dc_camp_tx=global, icoil_amp_camp_tx=global, icoil_rx_amp_err_camp_tx=global, vbat_camp_tx=global, vdc_camp_tx=global
  wires:
  Transfer Fcn4/1 -> Zero-Order Hold6/1  "ILB alias"
  Transfer Fcn3/1 -> Zero-Order Hold3/1  "ILA alias"
  Transfer Fcn1/1 -> Zero-Order Hold2/1
  Transfer Fcn/1 -> Zero-Order Hold1/1
  Zero-Order Hold8/1 -> [icoil_rx_amp_err_camp_tx]
  [icoil_rx_amp_err_radio_tx] -> Zero-Order Hold8/1
  Zero-Order Hold5/1 -> [icoil_amp_camp_tx], "icoil tx, icoil amp tx"/2
  Zero-Order Hold6/1 -> [i_leg_B_dc_dc_camp_tx]
  [i_leg_A_dc_dc_tx] -> Transfer Fcn3/1  "ILA"
  [i_leg_B_dc_dc_tx] -> Transfer Fcn4/1  "ILB"
  Zero-Order Hold3/1 -> [i_leg_A_dc_dc_camp_tx]
  [i_coil_tx] -> Abs2/1, "icoil tx, icoil amp tx"/1
  Zero-Order Hold2/1 -> [vbat_camp_tx]
  [v_bat_tx] -> Transfer Fcn1/1
  Zero-Order Hold1/1 -> [vdc_camp_tx]
  [v_dc_tx] -> Transfer Fcn/1
  Abs2/1 -> filtro PB/1
  filtro PB/1 -> Gain2/1
  [Stato_rx_radio_tx] -> Zero-Order Hold4/1
  Zero-Order Hold4/1 -> [Stato_rx_camp_tx]
  Gain2/1 -> "icoil tx, icoil amp tx"/3, Zero-Order Hold5/1

== system controllo_Completo_v14/Trasmissione radio (Ptrasf) ==
  note: Lato trasmettitore
  note: Questo scambio di dati avviene mentre si trasferisce potenza
      |  dal ricevitore (dx) al trasmettitore (sx)
  note: Questo scambio di dati avviene mentre si trasferisce potenza
      |  dal trasmettitore (sx) al ricevitore (dx)
  note: Lato ricevitore
  note: Questo scambio di dati avviene sempre
  Delay{1..6} (6 alike) : Delay  DelayLength=1  SampleTime=Ts_trasmissione
  Zero-Order Hold{1..6} (6 alike) : ZeroOrderHold  SampleTime=Ts_trasmissione
  tag scope: Ptrasf_rif_Vdc_rx_radio_tx=global, Ptrasf_rif_Vdc_tx_radio_rx=global, Stato_rx_radio_tx=global, Stato_tx_radio_rx=global, icoil_rx_amp_err_radio_tx=global, icoil_tx_amp_err_radio_rx=global
  wires:
  [icoil_tx_amp_err_tx] -> Delay5/1
  Zero-Order Hold1/1 -> [icoil_tx_amp_err_radio_rx]
  Zero-Order Hold3/1 -> [icoil_rx_amp_err_radio_tx]
  [icoil_rx_amp_err_rx] -> Delay4/1
  [Ptrasf_rif_Vdc_tx_tx] -> Delay2/1
  Zero-Order Hold4/1 -> [Ptrasf_rif_Vdc_tx_radio_rx]
  Zero-Order Hold5/1 -> [Ptrasf_rif_Vdc_rx_radio_tx]
  [Ptrasf_rif_Vdc_rx_rx] -> Delay3/1
  Delay2/1 -> Zero-Order Hold4/1
  Delay4/1 -> Zero-Order Hold3/1
  Delay3/1 -> Zero-Order Hold5/1
  Delay5/1 -> Zero-Order Hold1/1
  Delay1/1 -> Zero-Order Hold2/1
  [Stato_tx] -> Delay1/1
  Zero-Order Hold2/1 -> [Stato_tx_radio_rx]
  Delay6/1 -> Zero-Order Hold6/1
  [Stato_rx] -> Delay6/1
  Zero-Order Hold6/1 -> [Stato_rx_radio_tx]
